simulink model "CBF_for_Manipulator"  (R2024a)
settings: Solver=VariableStepAuto  StartTime=0.0  StopTime=Tf  RelTol=1e-3
undefined symbols (not defined in the file): InitPos, Ts, u_des
libraries: slctrl_constraint x1, robotmaniplib x1
settings Model: Creator=bumyong  LastModifiedBy=bumyong

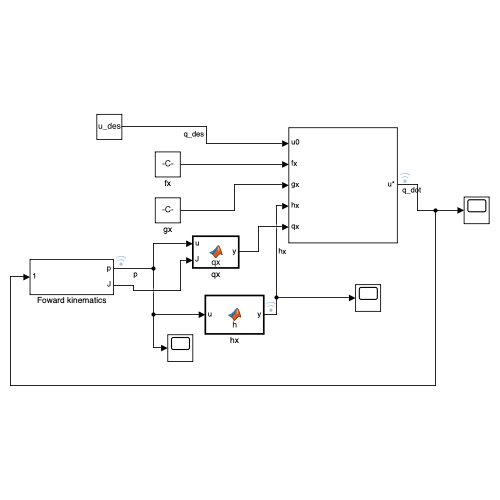
[thumbnail: Simulink's stored preview of the top-level diagram]
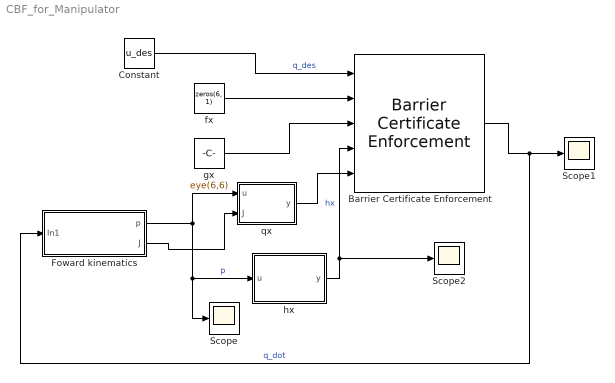
== system CBF_for_Manipulator ==
  Barrier Certificate Enforcement : slctrl_constraint/Barrier Certificate Enforcement  nx=6  nu=6  nc=1  gamma=gamma  beta=1  external_umax=off  external_umin=off  Ts=Ts  maxiter=200  tol=1e-6  output_exitflag=off
      settings: LibrarySourceBlock=slctrlblks/Constraint Control/Barrier Certificate Enforcement
  Constant : Constant  Value=u_des
  Foward kinematics : Subsystem
  Scope : Scope
  Scope1 : Scope
  Scope2 : Scope
  fx : Constant  Value=zeros(6, 1)
  gx : Constant  Value=eye(6,6)
  hx : MATLAB Function  TreatAsAtomicUnit=on
  qx : MATLAB Function  TreatAsAtomicUnit=on
  wires:
  Constant/1 -> Barrier Certificate Enforcement/1  "q_des"
  fx/1 -> Barrier Certificate Enforcement/2
  gx/1 -> Barrier Certificate Enforcement/3
  Barrier Certificate Enforcement/1 -> Foward kinematics/1(In1), Scope1/1  "q_dot"
  hx/1(y) -> Scope2/1, Barrier Certificate Enforcement/4  "hx"
  qx/1(y) -> Barrier Certificate Enforcement/5
  Foward kinematics/1(p) -> Scope/1, hx/1(u), qx/1(u)  "p"
  Foward kinematics/2(J) -> qx/2(J)

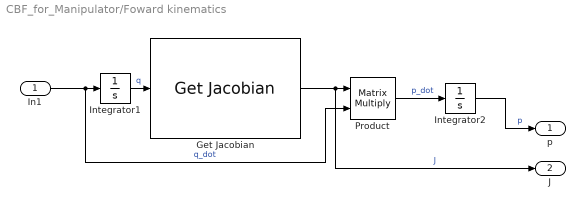
== system CBF_for_Manipulator/Foward kinematics ==
  In1 : Inport
  Get Jacobian : robotmaniplib/Get Jacobian  RigidBodyTree=robot  EndEffector=link7  SimulateUsing=Interpreted execution
  Integrator1 : Integrator
  Integrator2 : Integrator  InitialCondition=[0;0;0;InitPos]
  Product : Product  Multiplication=Matrix(*)
  p : Outport
  J : Outport  Port=2
  wires:
  Integrator1/1 -> Get Jacobian/1  "q"
  Product/1 -> Integrator2/1  "p_dot"
  In1/1 -> Product/2, Integrator1/1  "q_dot"
  Get Jacobian/1 -> J/1, Product/1  "J"
  Integrator2/1 -> p/1  "p"

== matlab function CBF_for_Manipulator/hx ==
  data: u input; y output
function y = h(u)

p = u(4:6);

R = 0.1;
R_w = 0.1;

p_obs = [0 0.4 1]';


y = norm(p - p_obs)^2 - (R + R_w)^2;

== matlab function CBF_for_Manipulator/qx ==
  data: u input; y output; J input
function y = qx(u, J)

p = u(4:6);
p_obs = [0 0.4 1]';



y = 2*(p-p_obs)'*J(4:6, :);
